simulink model "m06_linearization_model_MIMO"  (R2021a)
settings: Solver=VariableStepAuto  StartTime=0.0  StopTime=10  RelTol=1e-3
values from neighbouring files (symbols this model uses):
  a = L - b    (= 1.43208)    [m00_params.m]
  b = distr*L/(1 + distr)    (= 1.62792)    [m00_params.m]
  Cf = 1.205984111859764e+05    (= 120598.411186)    [m00_params.m]
  Cq = 8.888064374999998e+03    (= 8888.064375)    [m00_params.m]
  Cr = 1.117631261866039e+05    (= 111763.126187)    [m00_params.m]
  hs = 0.526    [m00_params.m]
  Ix = 850    [m00_params.m]
  Iz = 4600    [m00_params.m]
  Kq = 1.389290624725000e+05    (= 138929.062472)    [m00_params.m]
  M = 2500    [m00_params.m]
  ms = M - 2*mui    (= 2160)    [m00_params.m]
settings Model: Creator=jaime  LastModifiedBy=jason

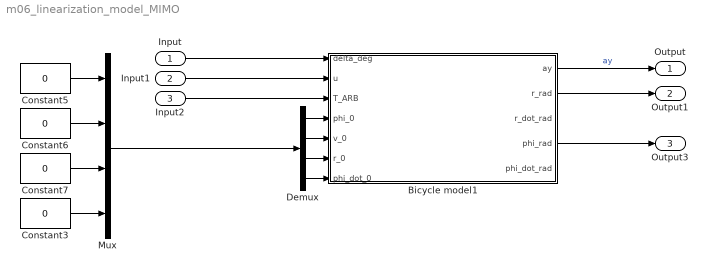
== system m06_linearization_model_MIMO ==
  Input : Inport
  Input1 : Inport  Port=2
  Input2 : Inport  Port=3
  Bicycle model1 : Subsystem
  Constant{3,5..7} (4 alike) : Constant  Value=0
  Demux : Demux
  Mux : Mux
  Output : Outport
  Output1 : Outport  Port=2
  Output3 : Outport  Port=3
  wires:
  Constant6/1 -> Mux/2
  Mux/1 -> Demux/1
  Constant7/1 -> Mux/3
  Constant5/1 -> Mux/1
  Constant3/1 -> Mux/4
  Demux/1 -> Bicycle model1/4(phi_0)
  Demux/2 -> Bicycle model1/5(v_0)
  Demux/3 -> Bicycle model1/6(r_0)
  Demux/4 -> Bicycle model1/7(phi_dot_0)
  Input/1 -> Bicycle model1/1(delta_deg)
  Input1/1 -> Bicycle model1/2(u)
  Input2/1 -> Bicycle model1/3(T_ARB)
  Bicycle model1/1(ay) -> Output/1  "ay"
  Bicycle model1/2(r_rad) -> Output1/1
  Bicycle model1/4(phi_rad) -> Output3/1

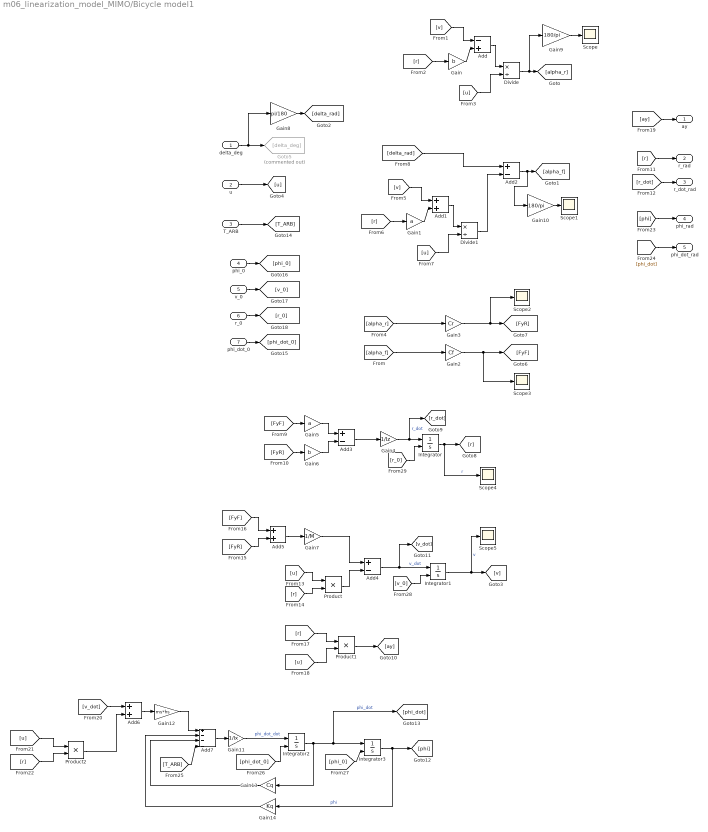
== system m06_linearization_model_MIMO/Bicycle model1 ==
  delta_deg : Inport
  u : Inport  Port=2
  T_ARB : Inport  Port=3
  phi_0 : Inport  Port=4
  v_0 : Inport  Port=5
  r_0 : Inport  Port=6
  phi_dot_0 : Inport  Port=7
  Add : Sum  Inputs=-+
  Add1 : Sum
  Add2 : Sum  Inputs=+-
  Add3 : Sum  Inputs=+-
  Add4 : Sum  Inputs=+-
  Add5 : Sum
  Add6 : Sum
  Add7 : Sum  Inputs=+---
  Divide : Product  Inputs=*/
  Divide1 : Product  Inputs=*/
  Gain : Gain  Gain=b
  Gain1 : Gain  Gain=a
  Gain10 : Gain  Gain=180/pi
  Gain11 : Gain  Gain=1/Ix
  Gain12 : Gain  Gain=ms*hs
  Gain13 : Gain  Gain=Cq
  Gain14 : Gain  Gain=Kq
  Gain2 : Gain  Gain=Cf
  Gain3 : Gain  Gain=Cr
  Gain4 : Gain  Gain=1/Iz
  Gain5 : Gain  Gain=a
  Gain6 : Gain  Gain=b
  Gain7 : Gain  Gain=1/M
  Gain8 : Gain  Gain=pi/180
  Gain9 : Gain  Gain=180/pi
  Goto5 : Goto  Commented=on  GotoTag=delta_deg
  Integrator{,1..3} (4 alike) : Integrator  InitialConditionSource=external
  Product : Product
  Product1 : Product
  Product2 : Product
  Scope{,1..5} (6 alike) : Scope
  ay : Outport
  r_rad : Outport  Port=2
  r_dot_rad : Outport  Port=3
  phi_rad : Outport  Port=4
  phi_dot_rad : Outport  Port=5
  wires:
  [v] -> Add/1
  [r] -> Gain/1
  Gain/1 -> Add/2
  u/1 -> [u]
  [u] -> Divide/2
  Add/1 -> Divide/1
  Divide/1 -> Gain9/1, [alpha_r]
  Gain1/1 -> Add1/2
  Add1/1 -> Divide1/1
  [r] -> Gain1/1
  [v] -> Add1/1
  [u] -> Divide1/2
  Add2/1 -> Gain10/1, [alpha_f]
  delta_deg/1 -> Gain8/1, Goto5/1
  [delta_rad] -> Add2/1
  Divide1/1 -> Add2/2
  Gain3/1 -> Scope2/1, [FyR]
  Gain2/1 -> Scope3/1, [FyF]
  [alpha_r] -> Gain3/1
  [alpha_f] -> Gain2/1
  Integrator/1 -> [r], Scope4/1  "r"
  Gain4/1 -> [r_dot], Integrator/1  "r_dot"
  [FyF] -> Gain5/1
  [FyR] -> Gain6/1
  Gain5/1 -> Add3/1
  Gain6/1 -> Add3/2
  Add3/1 -> Gain4/1
  [r] -> r_rad/1
  [r_dot] -> r_dot_rad/1
  Integrator1/1 -> Scope5/1, [v]  "v"
  Add4/1 -> [v_dot], Integrator1/1  "v_dot"
  [u] -> Product/1
  [r] -> Product/2
  Product/1 -> Add4/2
  [FyF] -> Add5/1
  [FyR] -> Add5/2
  Add5/1 -> Gain7/1
  Gain7/1 -> Add4/1
  [r] -> Product1/1
  [u] -> Product1/2
  Product1/1 -> [ay]
  [ay] -> ay/1
  Gain8/1 -> [delta_rad]
  Gain10/1 -> Scope1/1
  Gain9/1 -> Scope/1
  Integrator2/1 -> [phi_dot], Integrator3/1, Gain13/1  "phi_dot"
  Gain11/1 -> Integrator2/1  "phi_dot_dot"
  Integrator3/1 -> [phi], Gain14/1  "phi"
  [v_dot] -> Add6/1
  [u] -> Product2/1
  [r] -> Product2/2
  Product2/1 -> Add6/2
  Add6/1 -> Gain12/1
  Add7/1 -> Gain11/1
  Gain12/1 -> Add7/1
  Gain13/1 -> Add7/3
  Gain14/1 -> Add7/2
  [phi] -> phi_rad/1
  [phi_dot] -> phi_dot_rad/1
  T_ARB/1 -> [T_ARB]
  [T_ARB] -> Add7/4
  [phi_dot_0] -> Integrator2/2
  [phi_0] -> Integrator3/2
  [v_0] -> Integrator1/2
  [r_0] -> Integrator/2
  v_0/1 -> [v_0]
  r_0/1 -> [r_0]
  phi_0/1 -> [phi_0]
  phi_dot_0/1 -> [phi_dot_0]
